simulink model "greenmodel"  (R2014a)
settings: Solver=VariableStepAuto  StartTime=0.0  StopTime=15  RelTol=1e-3
libraries: simulink x1, CivilEnginelibV1 x1
settings Model: Creator=mmm  LastModifiedBy=mmm
settings DataIOCC: SaveFormat=Dataset
settings OptimizationCC: SimCompilerOptimization=off
settings DebuggingCC: MergeDetectMultiDrivingBlocksExec=error  SolverPrmCheckMsg=none  FrameProcessingCompatibilityMsg=error  AllowSymbolicDim=off
settings HardwareCC: ProdBitPerPointer=64  ProdLargestAtomicFloat=Float  ProdIntDivRoundTo=Zero  ProdEndianess=LittleEndian  ProdWordSize=64  ProdHWDeviceType=Intel->x86-64 (Windows64)
settings RTWCC: RTWCompilerOptimization=off
settings GRTTargetCC: GeneratePreprocessorConditionals=Use local settings
settings ConfigComp: CovMetricSettings=dw  CovHtmlReporting=on  CovSaveCumulativeToWorkspaceVar=on  CovSaveSingleToWorkspaceVar=on  CovExternalEMLEnable=off

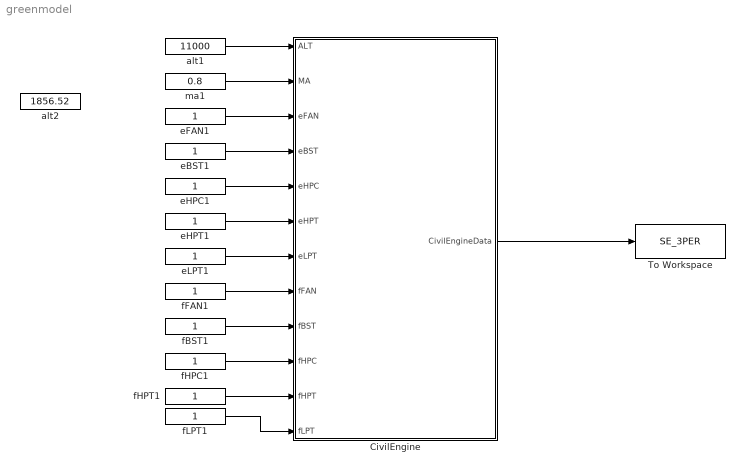
== system greenmodel ==
  CivilEngine : Subsystem
  To Workspace : ToWorkspace  VariableName=SE_3PER  SampleTime=-1
  alt1 : Constant  Value=11000
  alt2 : Constant  Value=1856.52
  eBST1 : Constant
  eFAN1 : Constant
  eHPC1 : Constant
  eHPT1 : Constant
  eLPT1 : Constant
  fBST1 : Constant
  fFAN1 : Constant
  fHPC1 : Constant
  fHPT1 : Constant
  fLPT1 : Constant
  ma1 : Constant  Value=0.8
  wires:
  CivilEngine/1(CivilEngineData) -> To Workspace/1
  alt1/1 -> CivilEngine/1(ALT)
  ma1/1 -> CivilEngine/2(MA)
  eFAN1/1 -> CivilEngine/3(eFAN)
  eBST1/1 -> CivilEngine/4(eBST)
  eHPC1/1 -> CivilEngine/5(eHPC)
  eHPT1/1 -> CivilEngine/6(eHPT)
  eLPT1/1 -> CivilEngine/7(eLPT)
  fFAN1/1 -> CivilEngine/8(fFAN)
  fBST1/1 -> CivilEngine/9(fBST)
  fHPC1/1 -> CivilEngine/10(fHPC)
  fHPT1/1 -> CivilEngine/11(fHPT)
  fLPT1/1 -> CivilEngine/12(fLPT)

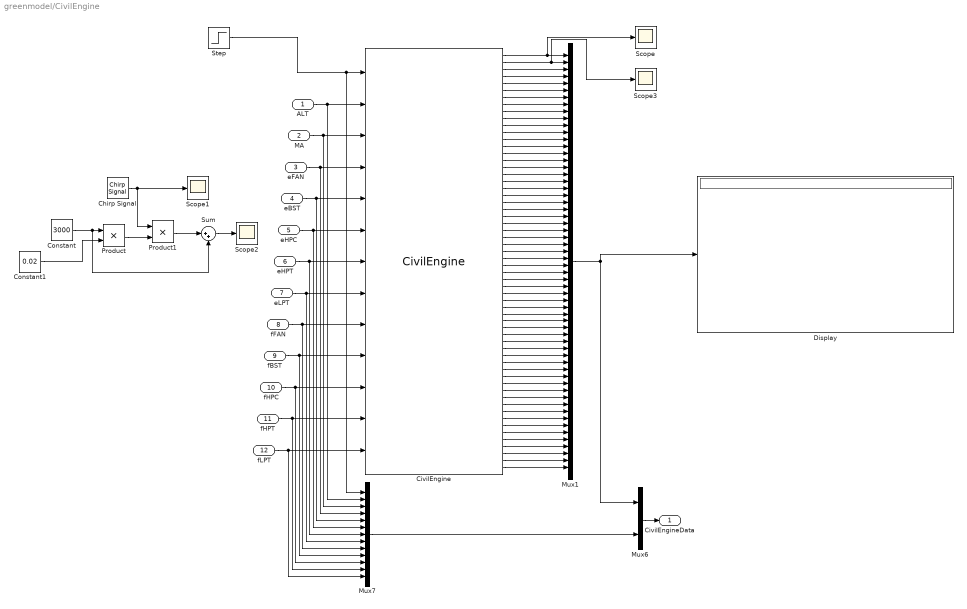
== system greenmodel/CivilEngine ==
  ALT : Inport
  MA : Inport  Port=2
  eFAN : Inport  Port=3
  eBST : Inport  Port=4
  eHPC : Inport  Port=5
  eHPT : Inport  Port=6
  eLPT : Inport  Port=7
  fFAN : Inport  Port=8
  fBST : Inport  Port=9
  fHPC : Inport  Port=10
  fHPT : Inport  Port=11
  fLPT : Inport  Port=12
  Chirp Signal : simulink/Sources/Chirp Signal  f1=0.1  T=15  f2=1
  CivilEngine : CivilEnginelibV1/CivilEngine  Initial_WF=1856.52  SampleTime=0.02  delta_T=0
  Constant : Constant  Value=3000
  Constant1 : Constant  Value=0.02
  Display : Display
  Mux1 : Mux  Inputs=60
  Mux6 : Mux  Inputs=2
  Mux7 : Mux  Inputs=13
  Product : Product
  Product1 : Product
  Scope{,1..3} (4 alike) : Scope
      Scope2 settings: SaveName=ScopeData2
  Step : Step  Before=1856.52  After=1856.52  SampleTime=0
  Sum : Sum  Inputs=|++
  CivilEngineData : Outport
  wires:
  Mux7/1 -> Mux6/2
  ALT/1 -> Mux7/2, CivilEngine/2
  MA/1 -> Mux7/3, CivilEngine/3
  eFAN/1 -> Mux7/4, CivilEngine/4
  eBST/1 -> Mux7/5, CivilEngine/5
  eHPC/1 -> Mux7/6, CivilEngine/6
  eHPT/1 -> Mux7/7, CivilEngine/7
  eLPT/1 -> Mux7/8, CivilEngine/8
  fFAN/1 -> Mux7/9, CivilEngine/9
  fBST/1 -> Mux7/10, CivilEngine/10
  fHPC/1 -> Mux7/11, CivilEngine/11
  fHPT/1 -> Mux7/12, CivilEngine/12
  fLPT/1 -> Mux7/13, CivilEngine/13
  CivilEngine/1 -> Scope/1, Mux1/1
  CivilEngine/2 -> Scope3/1, Mux1/2
  CivilEngine/3 -> Mux1/3
  CivilEngine/4 -> Mux1/4
  CivilEngine/5 -> Mux1/5
  CivilEngine/6 -> Mux1/6
  CivilEngine/7 -> Mux1/7
  CivilEngine/8 -> Mux1/8
  CivilEngine/9 -> Mux1/9
  CivilEngine/10 -> Mux1/10
  CivilEngine/11 -> Mux1/11
  CivilEngine/12 -> Mux1/12
  CivilEngine/13 -> Mux1/13
  CivilEngine/14 -> Mux1/14
  CivilEngine/15 -> Mux1/15
  CivilEngine/16 -> Mux1/16
  CivilEngine/17 -> Mux1/17
  CivilEngine/18 -> Mux1/18
  CivilEngine/19 -> Mux1/19
  CivilEngine/20 -> Mux1/20
  CivilEngine/21 -> Mux1/21
  CivilEngine/22 -> Mux1/22
  CivilEngine/23 -> Mux1/23
  CivilEngine/24 -> Mux1/24
  CivilEngine/25 -> Mux1/25
  CivilEngine/26 -> Mux1/26
  CivilEngine/27 -> Mux1/27
  CivilEngine/28 -> Mux1/28
  CivilEngine/29 -> Mux1/29
  CivilEngine/30 -> Mux1/30
  CivilEngine/31 -> Mux1/31
  CivilEngine/32 -> Mux1/32
  CivilEngine/33 -> Mux1/33
  CivilEngine/34 -> Mux1/34
  CivilEngine/35 -> Mux1/35
  CivilEngine/36 -> Mux1/36
  CivilEngine/37 -> Mux1/37
  CivilEngine/38 -> Mux1/38
  CivilEngine/39 -> Mux1/39
  CivilEngine/40 -> Mux1/40
  CivilEngine/41 -> Mux1/41
  CivilEngine/42 -> Mux1/42
  CivilEngine/43 -> Mux1/43
  CivilEngine/44 -> Mux1/44
  CivilEngine/45 -> Mux1/45
  CivilEngine/46 -> Mux1/46
  CivilEngine/47 -> Mux1/47
  CivilEngine/48 -> Mux1/48
  CivilEngine/49 -> Mux1/49
  CivilEngine/50 -> Mux1/50
  CivilEngine/51 -> Mux1/51
  CivilEngine/52 -> Mux1/52
  CivilEngine/53 -> Mux1/53
  CivilEngine/54 -> Mux1/54
  CivilEngine/55 -> Mux1/55
  CivilEngine/56 -> Mux1/56
  CivilEngine/57 -> Mux1/57
  CivilEngine/58 -> Mux1/58
  CivilEngine/59 -> Mux1/59
  CivilEngine/60 -> Mux1/60
  Mux1/1 -> Mux6/1, Display/1
  Mux6/1 -> CivilEngineData/1
  Chirp Signal/1 -> Product1/1, Scope1/1
  Constant1/1 -> Product/2
  Product/1 -> Product1/2
  Product1/1 -> Sum/1
  Constant/1 -> Sum/2, Product/1
  Sum/1 -> Scope2/1
  Step/1 -> CivilEngine/1, Mux7/1
